simulink model "lab3Mod"  (Simulink 4.00)
settings: Solver=ode45  SolverMode=SingleTasking  StartTime=0.0  StopTime=9999  MaxStep=.01  RelTol=1e-3  AbsTol=1e-6
libraries: simulink3 x1
settings Model: Creator=vise  LastModifiedBy=vise  LimitDataPoints=off  RTWTemplateMakefile=grt_unix.tmf  ExtModeTrigMode=oneshot  ExtModeArmWhenConnect=off  ExtModeAutoUpdateStatusClock=off

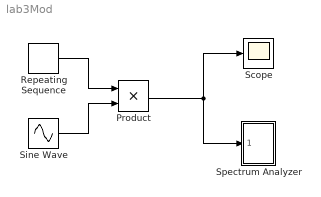
== system lab3Mod ==
  Product : Product  Inputs=2  Multiplication=Element-wise(.*)  SaturateOnIntegerOverflow=on
  Repeating Sequence : simulink3/Sources/Repeating Sequence  rep_seq_t=[0 0.5 1 2]  rep_seq_y=[0 1 0 0]
  Scope : Scope
      settings: TickLabels=on  TimeRange=10  YMin=-1.5  YMax=1.5  SaveToWorkspace=off  SaveName=ScopeData  DataFormat=Array  LimitDataPoints=on  MaxDataPoints=5000
  Sine Wave : Sin  SineType=Time-based  Amplitude=1  Bias=0  Frequency=2*pi*10  Phase=0  Samples=10  SampleTime=0  Offset=0
  Spectrum Analyzer : Subsystem  mask(Spectrum analyzer.){@1=2048, @2=0.02, @3=10}
      mask prompts: @1 "Number of sample points:"; @2 "Sampling period (sec):"; @3 "Plotting Period (sec):"
      mask init:
      | N=@1; T_s=@2;plot_period=@3;
      settings: RTWFcnNameOpts=Auto  RTWFileNameOpts=Auto
      mask Help: EE438 Lab utility; See Prof. Bouman.
      mask Display: plot(0,0,100,100,[14,91,91,14,14],[86,86,40,40,86],[85,82,80,79,75,67,63,60,57,53,41,36,33,27,24],[49,50,53,50,49,51,54,66,54,50,50,52,81,51,49])
  wires:
  Product/1 -> Spectrum Analyzer/1(input signal), Scope/1
  Repeating Sequence/1 -> Product/1
  Sine Wave/1 -> Product/2

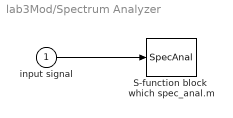
== system lab3Mod/Spectrum Analyzer ==
  input signal : Inport  Port=1  LatchInput=off
  S-function block  which spec_anal.m : S-Function  FunctionName=SpecAnal  Parameters=N,T_s,plot_period  PortCounts=[]  SFunctionModules=''
  wires:
  input signal/1 -> S-function block  which spec_anal.m/1
